simulink model "asim"  (R2023a)
settings: Solver=FixedStepDiscrete  StartTime=0.0  StopTime=10.0  RelTol=1e-3
libraries: simulink x2
settings Model: Creator=u29w13  LastModifiedBy=u29w13

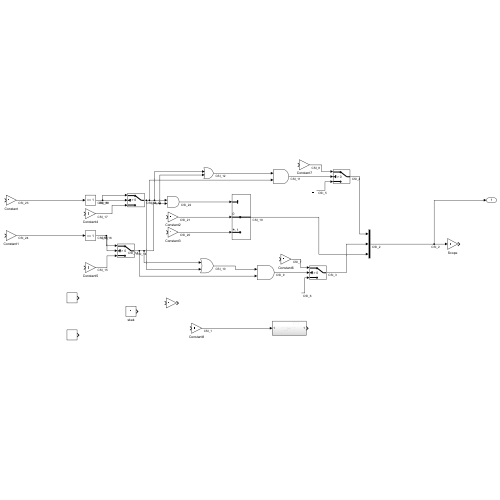
[thumbnail: Simulink's stored preview of the top-level diagram]
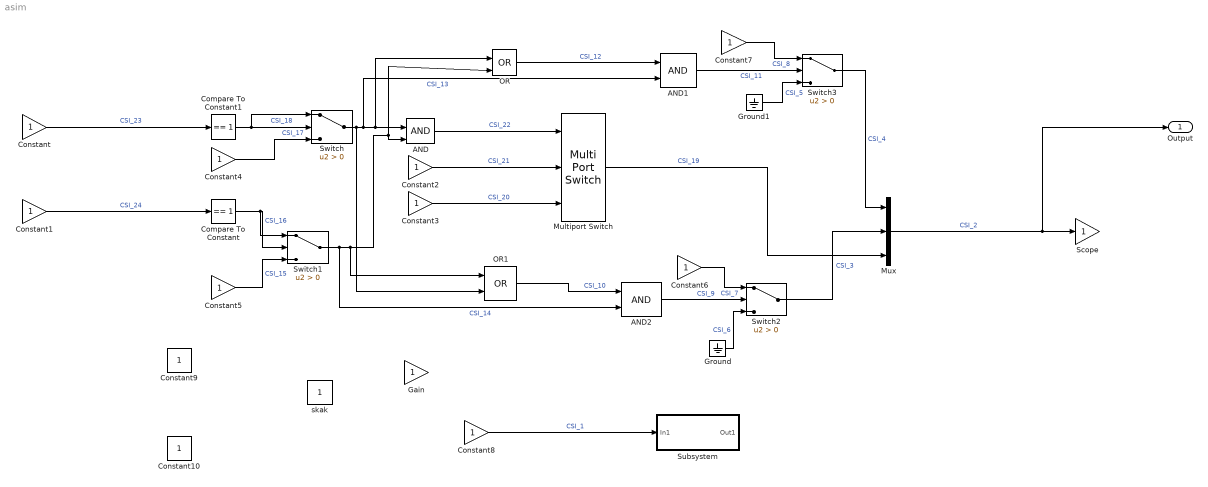
== system asim ==
  AND : Logic  IconShape=distinctive  AllPortsSameDT=off  OutDataTypeStr=boolean
  AND1 : Logic  IconShape=distinctive  AllPortsSameDT=off  OutDataTypeStr=boolean
  AND2 : Logic  IconShape=distinctive  AllPortsSameDT=off  OutDataTypeStr=boolean
  Compare To Constant : simulink/Logic and Bit Operations/Compare To Constant  relop===  const=1  OutDataTypeStr=boolean
  Compare To Constant1 : simulink/Logic and Bit Operations/Compare To Constant  relop===  const=1  OutDataTypeStr=boolean
  Constant{,1..8} (9 alike) : Gain
  Constant10 : Constant
  Constant9 : Constant
  Gain : Gain
  Ground : Ground
  Ground1 : Ground
  Multiport Switch : MultiPortSwitch  DataPortOrder=Zero-based contiguous  Inputs=2  zeroidx=on  SaturateOnIntegerOverflow=off  InputSameDT=off
  Mux : Mux  Inputs=3
  OR : Logic  Operator=OR  IconShape=distinctive  AllPortsSameDT=off  OutDataTypeStr=boolean
  OR1 : Logic  Operator=OR  IconShape=distinctive  AllPortsSameDT=off  OutDataTypeStr=boolean
  Scope : Gain
  Subsystem : Subsystem
  Switch{,1..3} (4 alike) : Switch  Criteria=u2 > Threshold  SaturateOnIntegerOverflow=off  InputSameDT=off
  skak : Constant
  Output : Outport
  wires:
  Constant1/1 -> Compare To Constant/1  "CSI_24"
  Constant/1 -> Compare To Constant1/1  "CSI_23"
  AND/1 -> Multiport Switch/1  "CSI_22"
  Constant2/1 -> Multiport Switch/2  "CSI_21"
  Constant3/1 -> Multiport Switch/3  "CSI_20"
  Multiport Switch/1 -> Mux/3  "CSI_19"
  Compare To Constant1/1 -> Switch/1, Switch/2  "CSI_18"
  Constant4/1 -> Switch/3  "CSI_17"
  Compare To Constant/1 -> Switch1/1, Switch1/2  "CSI_16"
  Constant5/1 -> Switch1/3  "CSI_15"
  Switch1/1 -> OR/2, AND/2, OR1/1, AND2/2  "CSI_14"
  Switch/1 -> OR1/2, AND1/2, OR/1, AND/1  "CSI_13"
  OR/1 -> AND1/1  "CSI_12"
  AND1/1 -> Switch3/2  "CSI_11"
  OR1/1 -> AND2/1  "CSI_10"
  AND2/1 -> Switch2/2  "CSI_9"
  Constant7/1 -> Switch3/1  "CSI_8"
  Constant6/1 -> Switch2/1  "CSI_7"
  Ground/1 -> Switch2/3  "CSI_6"
  Ground1/1 -> Switch3/3  "CSI_5"
  Switch3/1 -> Mux/1  "CSI_4"
  Switch2/1 -> Mux/2  "CSI_3"
  Mux/1 -> Output/1, Scope/1  "CSI_2"
  Constant8/1 -> Subsystem/1(In1)  "CSI_1"

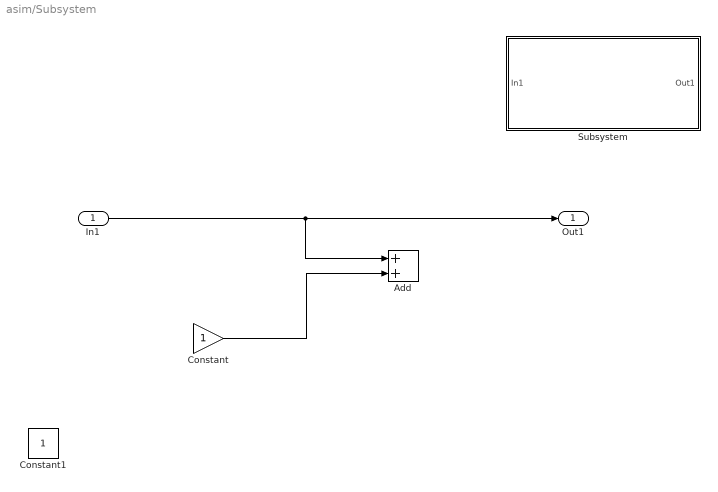
== system asim/Subsystem ==
  In1 : Inport
  Add : Sum
  Constant : Gain
  Constant1 : Constant
  Subsystem : Subsystem
  Out1 : Outport
  wires:
  In1/1 -> Add/1, Out1/1
  Constant/1 -> Add/2

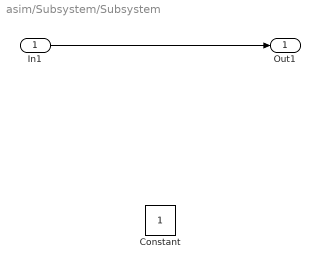
== system asim/Subsystem/Subsystem ==
  In1 : Inport
  Constant : Constant
  Out1 : Outport
  wires:
  In1/1 -> Out1/1
